simulink model "s_pol1"  (Simulink 8.1)
settings: Solver=ode45  SolverMode=SingleTasking  StartTime=0.0  StopTime=50  MaxStep=0.10  RelTol=1e-3  AbsTol=1e-6
values from neighbouring files (symbols this model uses):
  k1 = K(1)    [alqr1.m]    (also in alqrd1.m; apol1.m; pol1.m = -2*a*T1-1-T1/T2; pol2.m = -2*a*T1-1-T1/T2)
  k2 = K(2)    [alqr1.m]    (also in alqrd1.m; apol1.m; pol1.m = (a^2+b^2)*T1*T2-1-k1; pol2.m = (a^2+b^2)*T1*T2-1-k1)
  T1 = -5    [pol1.m]    (also in pol2.m; pol3.m; pol4.m)
  T2 = 10    [pol1.m]    (also in pol2.m; pol3.m; pol4.m)
  x10 = 1    [pol1.m]
  x20 = 0    [pol1.m]
libraries: simulink x2
settings Model: Creator=mainster  LastModifiedBy=mainster
settings DataIOCC: LimitDataPoints=off  SaveOutput=off  SaveTime=off
settings OptimizationCC: BlockReduction=off  BooleanDataType=off  ExpressionDepthLimit=128
settings DebuggingCC: SaveWithParameterizedLinksMsg=none  SignalResolutionControl=TryResolveAllWithWarning  SolverPrmCheckMsg=none  MultiTaskDSMMsg=warning  MultiTaskCondExecSysMsg=none  FcnCallInpInsideContextMsg=EnableAllAsError  StrictBusMsg=None
settings HardwareCC: TargetUnknown=on
settings RTWCC: IncludeERTFirstTime=on

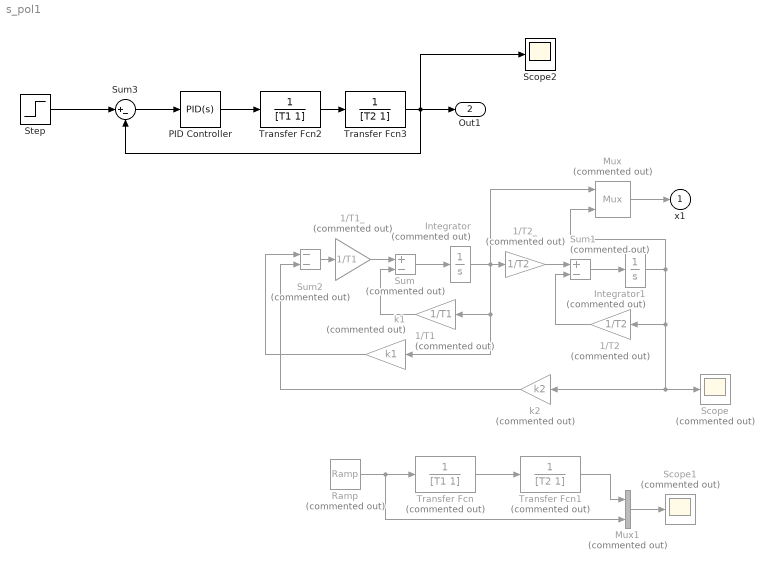
== system s_pol1 ==
  1/T1 : Gain  Commented=on  Gain=1/T1  SaturateOnIntegerOverflow=on  OutDataTypeStr=Inherit: Same as input  ParamDataTypeStr=Inherit: Same as input
  1/T1_ : Gain  Commented=on  Gain=1/T1  SaturateOnIntegerOverflow=on  OutDataTypeStr=Inherit: Same as input  ParamDataTypeStr=Inherit: Same as input
  1/T2 : Gain  Commented=on  Gain=1/T2  SaturateOnIntegerOverflow=on  OutDataTypeStr=Inherit: Same as input  ParamDataTypeStr=Inherit: Same as input
  1/T2_ : Gain  Commented=on  Gain=1/T2  SaturateOnIntegerOverflow=on  OutDataTypeStr=Inherit: Same as input  ParamDataTypeStr=Inherit: Same as input
  Integrator : Integrator  Commented=on  InitialCondition=x10
  Integrator1 : Integrator  Commented=on  InitialCondition=x20
  Mux : Mux  Commented=on  Inputs=2
  Mux1 : Mux  Commented=on  Inputs=2
  PID Controller : simulink/Continuous/PID Controller  Controller=PID  TimeDomain=Continuous-time  SampleTime=1  IntegratorMethod=Forward Euler  FilterMethod=Forward Euler  Form=Parallel  P=-38.4773563906226  I=-1.01032339760756  D=-191.402598783563  N=7.54131822931917  InitialConditionSource=internal  InitialConditionForIntegrator=0  InitialConditionForFilter=0  ExternalReset=none  LimitOutput=off  UpperSaturationLimit=inf  LowerSaturationLimit=-inf  LinearizeAsGain=on  AntiWindupMode=none  Kb=1  TrackingMode=off  Kt=1  PParamMin=[]  PParamMax=[]  IParamMin=[]  IParamMax=[]  DParamMin=[]  DParamMax=[]  NParamMin=[]  NParamMax=[]  KbParamMin=[]  KbParamMax=[]  KtParamMin=[]  KtParamMax=[]  POutMin=[]  POutMax=[]  IOutMin=[]  IOutMax=[]  DOutMin=[]  DOutMax=[]  NOutMin=[]  NOutMax=[]  KbOutMin=[]  KbOutMax=[]  KtOutMin=[]  KtOutMax=[]  IntegratorOutMin=[]  IntegratorOutMax=[]  FilterOutMin=[]  FilterOutMax=[]  SumOutMin=[]  SumOutMax=[]  SumI1OutMin=[]  SumI1OutMax=[]  SumI2OutMin=[]  SumI2OutMax=[]  SumI3OutMin=[]  SumI3OutMax=[]  SumDOutMin=[]  SumDOutMax=[]  SaturationOutMin=[]  SaturationOutMax=[]  IntegratorContinuousStateAttributes=''  IntegratorStateMustResolveToSignalObject=off  IntegratorRTWStateStorageClass=Auto  FilterContinuousStateAttributes=''  FilterStateMustResolveToSignalObject=off  FilterRTWStateStorageClass=Auto
  Ramp : simulink/Sources/Ramp  Commented=on  slope=50  start=0  X0=0
  Scope : Scope  Commented=on
      settings: TickLabels=on  TimeRange=50.000000  YMin=-1.540000  YMax=1.540000
  Scope1 : Scope  Commented=on
      settings: TickLabels=on  TimeRange=50.000000  YMin=-1.540000  YMax=1.540000
  Scope2 : Scope
      settings: SaveName=ScopeData2
  Step : Step  SampleTime=0
  Sum : Sum  Commented=on  Inputs=+-  SaturateOnIntegerOverflow=on  InputSameDT=on  OutDataTypeStr=Inherit: Same as first input
  Sum1 : Sum  Commented=on  Inputs=+-  SaturateOnIntegerOverflow=on  InputSameDT=on  OutDataTypeStr=Inherit: Same as first input
  Sum2 : Sum  Commented=on  Inputs=--  SaturateOnIntegerOverflow=on  InputSameDT=on  OutDataTypeStr=Inherit: Same as first input
  Sum3 : Sum  Inputs=|+-
  Transfer Fcn : TransferFcn  Commented=on  Denominator=[T1 1]
  Transfer Fcn1 : TransferFcn  Commented=on  Denominator=[T2 1]
  Transfer Fcn2 : TransferFcn  Denominator=[T1 1]
  Transfer Fcn3 : TransferFcn  Denominator=[T2 1]
  k1 : Gain  Commented=on  Gain=k1  SaturateOnIntegerOverflow=on  OutDataTypeStr=Inherit: Same as input  ParamDataTypeStr=Inherit: Same as input
  k2 : Gain  Commented=on  Gain=k2  SaturateOnIntegerOverflow=on  OutDataTypeStr=Inherit: Same as input  ParamDataTypeStr=Inherit: Same as input
  x1 : Outport  InitialOutput=0
  Out1 : Outport  Port=2
  wires:
  Mux/1 -> x1/1
  Integrator1/1 -> Scope/1, k2/1, 1/T2/1, Mux/2
  k2/1 -> Sum2/2
  k1/1 -> Sum2/1
  Sum2/1 -> 1/T1_/1
  Integrator/1 -> k1/1, 1/T1/1, Mux/1, 1/T2_/1
  Sum1/1 -> Integrator1/1
  1/T2/1 -> Sum1/2
  1/T2_/1 -> Sum1/1
  Sum/1 -> Integrator/1
  1/T1/1 -> Sum/2
  1/T1_/1 -> Sum/1
  Transfer Fcn/1 -> Transfer Fcn1/1
  Transfer Fcn1/1 -> Mux1/1
  Ramp/1 -> Mux1/2, Transfer Fcn/1
  Mux1/1 -> Scope1/1
  Transfer Fcn2/1 -> Transfer Fcn3/1
  PID Controller/1 -> Transfer Fcn2/1
  Sum3/1 -> PID Controller/1
  Transfer Fcn3/1 -> Scope2/1, Sum3/2, Out1/1
  Step/1 -> Sum3/1
